simulink model "linear_ss_control_with_reference"  (R2019b)
settings: Solver=ode45  StartTime=0.0  StopTime=700  MaxStep=0.001  RelTol=1e-8
settings Model: Creator=Hector  LastModifiedBy=Hector

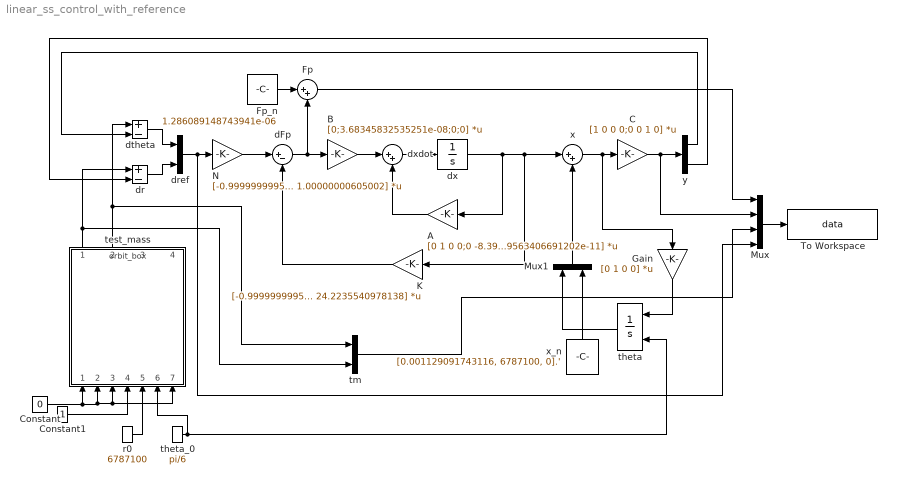
== system linear_ss_control_with_reference ==
  A : Gain  Gain=[0 1 0 0;0 -8.39126813382404e-11 -1.39595873998803e-20 -3.3271699050138e-10;0 0 0 1;0 15326.5171394046 3.8245444931179e-06 -4.19563406691202e-11]  Multiplication=Matrix(K*u)
  B : Gain  Gain=[0;3.68345832535251e-08;0;0]  Multiplication=Matrix(K*u)
  C : Gain  Gain=[1 0 0 0;0 0 1 0]  Multiplication=Matrix(K*u)
  Constant : Constant  Value=0
  Constant1 : Constant
  Fp : Sum  Inputs=|++
  Fp_n : Constant  Value=1.286089148743941e-06
  Gain : Gain  Gain=[0 1 0 0]  Multiplication=Matrix(K*u)
  K : Gain  Gain=[-0.999999999517925 4489802.13130477 1.00112038113525 24.2235540978138]  Multiplication=Matrix(K*u)
  Mux : Mux
  Mux1 : Mux  Inputs=2
  N : Gain  Gain=[-0.999999999517925 1.00000000605002]  Multiplication=Matrix(K*u)
  To Workspace : ToWorkspace  VariableName=data  SaveFormat=Timeseries  SampleTime=-1
  dFp : Sum  Inputs=|+-
  dr : Sum  Inputs=+-
  dref : Mux  Inputs=2
  dtheta : Sum  Inputs=+-
  dx : Integrator  InitialCondition=[0, 0, -1*10^-6, 0].'
  dxdot : Sum  Inputs=|++
  r0 : Constant  Value=6787100
  test_mass : ModelReference  ModelNameDialog=orbit_box.slx  SimulationMode=Normal  ModelReferenceVersion=1.38
  theta : Integrator  InitialConditionSource=external
  theta_0 : Constant  Value=pi/6
  tm : Mux  Inputs=2
  x : Sum  Inputs=|++
  x_n : Constant  Value=[0.001129091743116, 6787100, 0].'
  y : Demux  Outputs=2
  wires:
  Fp_n/1 -> Fp/1
  dxdot/1 -> dx/1
  N/1 -> dFp/1
  Fp/1 -> Mux/1
  A/1 -> dxdot/2
  dref/1 -> Mux/4, N/1
  C/1 -> Mux/2, y/1
  K/1 -> dFp/2
  x/1 -> Gain/1, C/1
  B/1 -> dxdot/1
  dx/1 -> x/1, K/1, A/1
  dFp/1 -> B/1, Fp/2
  dtheta/1 -> dref/1
  dr/1 -> dref/2
  test_mass/1 -> dr/1, tm/2
  test_mass/2 -> tm/1, dtheta/1
  y/2 -> dr/2
  y/1 -> dtheta/2
  Constant/1 -> test_mass/1, test_mass/7, test_mass/3, test_mass/2
  Gain/1 -> theta/1
  theta/1 -> Mux1/1
  Mux1/1 -> x/2
  x_n/1 -> Mux1/2
  Constant1/1 -> test_mass/4
  theta_0/1 -> test_mass/6, theta/2
  r0/1 -> test_mass/5
  tm/1 -> Mux/3
  Mux/1 -> To Workspace/1
